simulink model "Verifica_EIG_11032026"  (R2025b)
settings: Solver=VariableStepAuto  StartTime=0.0  StopTime=20.0  RelTol=1e-3
values from neighbouring files (symbols this model uses):
  A = double(subs(A_sym, x, x_star))    [SvolgimentoEsame_11032026.m]
  B = double(subs(B_sym, x, x_star))    [SvolgimentoEsame_11032026.m]
  N = -inv(C_N * (A_cl \ B))    [SvolgimentoEsame_11032026.m]
undefined symbols (not defined in the file or in its folder): C_eig, D_eig, K_EIG, q0, q_ref
settings Model: Creator=salvo  LastModifiedBy=salvo

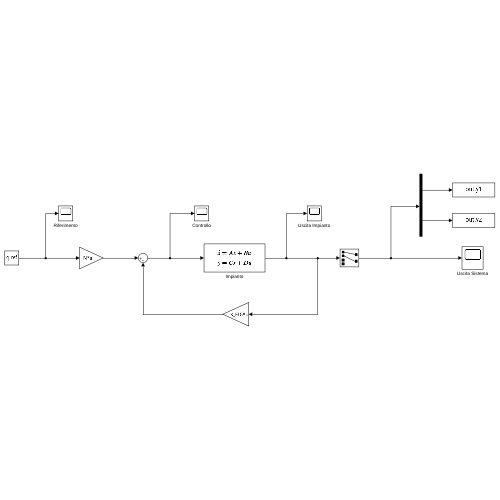
[thumbnail: Simulink's stored preview of the top-level diagram]
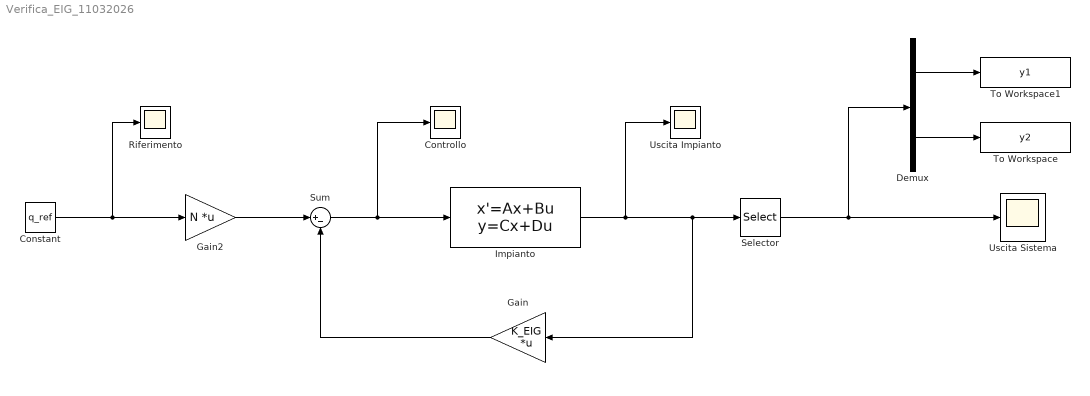
== system Verifica_EIG_11032026 ==
  Constant : Constant  Value=q_ref
  Controllo : Scope
      settings: DataLoggingVariableName=ScopeData2
  Demux : Demux  Outputs=2
  Gain : Gain  Gain=K_EIG  Multiplication=Matrix(K*u)
  Gain2 : Gain  Gain=N  Multiplication=Matrix(K*u)
  Impianto : StateSpace  A=A  B=B  C=C_eig  D=D_eig  InitialCondition=q0
  Riferimento : Scope
  Selector : Selector  InputPortWidth=4  IndexOptions=Index vector (dialog)  Indices=[1 2]  OutputSizes=1
  Sum : Sum  Inputs=|+-
  To Workspace : ToWorkspace  VariableName=y2  SaveFormat=Timeseries  SampleTime=-1
  To Workspace1 : ToWorkspace  VariableName=y1  SaveFormat=Timeseries  SampleTime=-1
  Uscita Impianto : Scope
      settings: DataLoggingVariableName=ScopeData3
  Uscita Sistema : Scope
      settings: ActiveDisplayYMinimum=-0.24936092619821471  ActiveDisplayYMaximum=1.0421108235964467
  wires:
  Sum/1 -> Impianto/1, Controllo/1
  Gain/1 -> Sum/2
  Impianto/1 -> Selector/1, Gain/1, Uscita Impianto/1
  Constant/1 -> Riferimento/1, Gain2/1
  Gain2/1 -> Sum/1
  Selector/1 -> Demux/1, Uscita Sistema/1
  Demux/1 -> To Workspace1/1
  Demux/2 -> To Workspace/1
